simulink model "Master_Robot"  (R2019b)
settings: Solver=VariableStepAuto  StartTime=0.0  StopTime=10  RelTol=1e-3
undefined symbols (not defined in the file): Bh, Bs, Fc_h, Jh, k_m, Kc2v_m, Kd_h, Kd_s, Kp_h, Kp_s, Ks, Kt2c_m, lArm_m, maxCurrent_m, tau_s
settings Model: Creator=Mirko  LastModifiedBy=Mirko
settings SFSimCC: CustomCodeUndefinedFunction=UseInterfaceOnly

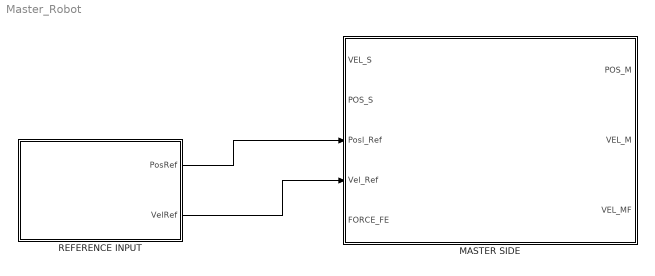
== system Master_Robot ==
  MASTER SIDE : Subsystem
  REFERENCE INPUT : Subsystem
  wires:
  REFERENCE INPUT/1(PosRef) -> MASTER SIDE/3(Posl_Ref)
  REFERENCE INPUT/2(VelRef) -> MASTER SIDE/4(Vel_Ref)

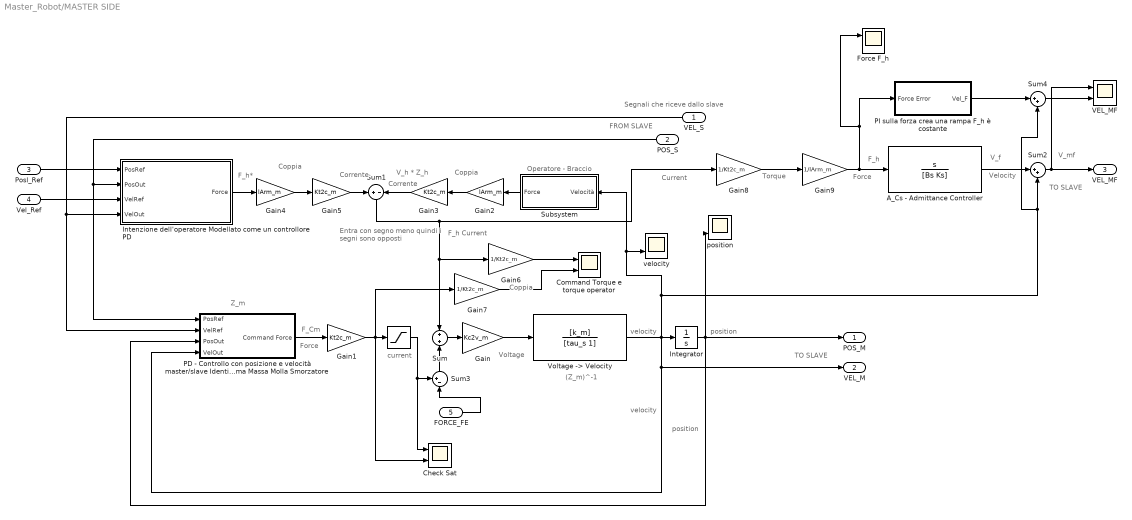
== system Master_Robot/MASTER SIDE ==
  note: Velocity
  note: Force
  note: Torque
  note: Current
  note: V_mf
  note: V_f
  note: F_h
  note: Z_m
  note: (Z_m)^-1
  note: F_h Current
  note: V_h * Z_h
  note: F_h*
  note: F_Cm
  note: FROM SLAVE
  note: TO SLAVE
  note: Coppia
  note: Entra con segno meno quindi
      | i segni sono opposti
  note: Corrente
  note: Coppia
  note: Corrente
  note: Coppia
  note: Segnali che riceve dallo slave
  note: Operatore - Braccio
  note: current
  note: Force
  note: Voltage
  note: position
  note: velocity
  note: position
  note: velocity
  note: TO SLAVE
  "VEL_S " : Inport
  POS_S : Inport  Port=2
  Posl_Ref : Inport  Port=3
  Vel_Ref : Inport  Port=4
  "FORCE_FE " : Inport  Port=5
  " " : Saturate  UpperLimit=maxCurrent_m  LowerLimit=-maxCurrent_m
  A_Cs - Admittance Controller : TransferFcn  Numerator=[1 0]  Denominator=[Bs Ks]
  Check Sat : Scope  NumInputPorts=2
  "Command Torque e torque operator " : Scope  NumInputPorts=2
  "Force F_h " : Scope  NumInputPorts=2
  Gain : Gain  Gain=Kc2v_m
  Gain1 : Gain  Gain=Kt2c_m
  Gain2 : Gain  Gain=lArm_m
  Gain3 : Gain  Gain=Kt2c_m
  Gain4 : Gain  Gain=lArm_m
  Gain5 : Gain  Gain=Kt2c_m
  Gain6 : Gain  Gain=1/Kt2c_m
  Gain7 : Gain  Gain=1/Kt2c_m
  Gain8 : Gain  Gain=1/Kt2c_m
  Gain9 : Gain  Gain=1/lArm_m
  Integrator : Integrator
  Intenzione dell'operatore Modellato come un controllore PD : Subsystem
  PD - Controllo con posizione e velocità master/slave Identico all'accoppiamento virtuale Sistema Massa Molla Smorzatore : Subsystem
  "PI sulla forza crea una rampa F_h è costante " : Subsystem
  Subsystem : Subsystem
  Sum : Sum
  Sum1 : Sum  Inputs=+-
  Sum2 : Sum  Inputs=|++
  Sum3 : Sum  Inputs=+-|
  Sum4 : Sum  Inputs=|++
  "VEL_MF " : Scope  NumInputPorts=2
  "Voltage -> Velocity " : TransferFcn  Numerator=[k_m]  Denominator=[tau_s 1]
  position : Scope  NumInputPorts=2
  velocity : Scope  NumInputPorts=2
  POS_M : Outport
  VEL_M : Outport  Port=2
  VEL_MF : Outport  Port=3
  wires:
  Gain1/1 -> Gain7/1, Check Sat/2, " "/1
  "VEL_S "/1 -> PD - Controllo con posizione e velocità master/slave Identico all'accoppiamento virtuale Sistema Massa Molla Smorzatore/2(VelRef), Intenzione dell'operatore Modellato come un controllore PD/4(VelOut)
  Integrator/1 -> PD - Controllo con posizione e velocità master/slave Identico all'accoppiamento virtuale Sistema Massa Molla Smorzatore/3(PosOut), position/2, POS_M/1
  ? -> position/1
  "Voltage -> Velocity "/1 -> PD - Controllo con posizione e velocità master/slave Identico all'accoppiamento virtuale Sistema Massa Molla Smorzatore/4(VelOut), VEL_M/1, Integrator/1, Sum4/2, Sum2/2, Subsystem/1("Velocità "), velocity/2
  Sum1/1 -> Gain8/1, Gain6/1, Sum/1
  Gain4/1 -> Gain5/1
  Gain6/1 -> "Command Torque e torque operator "/1
  Subsystem/1(Force) -> Gain2/1
  POS_S/1 -> Intenzione dell'operatore Modellato come un controllore PD/2(PosOut), PD - Controllo con posizione e velocità master/slave Identico all'accoppiamento virtuale Sistema Massa Molla Smorzatore/1(PosRef)
  Gain2/1 -> Gain3/1
  PD - Controllo con posizione e velocità master/slave Identico all'accoppiamento virtuale Sistema Massa Molla Smorzatore/1("Command Force ") -> Gain1/1
  Gain3/1 -> Sum1/2
  Gain7/1 -> "Command Torque e torque operator "/2
  Gain5/1 -> Sum1/1
  " "/1 -> Check Sat/1, Sum3/1
  ? -> velocity/1
  Intenzione dell'operatore Modellato come un controllore PD/1("Force ") -> Gain4/1
  Gain/1 -> "Voltage -> Velocity "/1
  Sum/1 -> Gain/1
  Posl_Ref/1 -> Intenzione dell'operatore Modellato come un controllore PD/1("PosRef ")
  Vel_Ref/1 -> Intenzione dell'operatore Modellato come un controllore PD/3(VelRef)
  A_Cs - Admittance Controller/1 -> Sum2/1
  Sum2/1 -> "VEL_MF "/1, VEL_MF/1
  "FORCE_FE "/1 -> Sum3/2
  Sum3/1 -> Sum/2
  Gain8/1 -> Gain9/1
  Gain9/1 -> "Force F_h "/1, "PI sulla forza crea una rampa F_h è costante "/1("Force Error "), A_Cs - Admittance Controller/1
  "PI sulla forza crea una rampa F_h è costante "/1(Vel_F) -> Sum4/1
  Sum4/1 -> "VEL_MF "/2

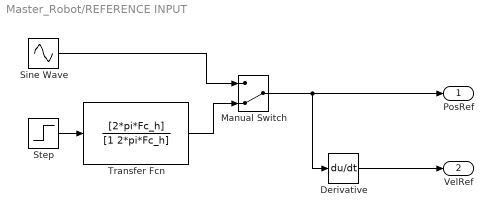
== system Master_Robot/REFERENCE INPUT ==
  Derivative : Derivative
  Manual Switch : ManualSwitch  CurrentSetting=0
  Sine Wave : Sin  SampleTime=0
  Step : Step  SampleTime=0
  Transfer Fcn : TransferFcn  Numerator=[2*pi*Fc_h]  Denominator=[1 2*pi*Fc_h]
  PosRef : Outport
  VelRef : Outport  Port=2
  wires:
  Sine Wave/1 -> Manual Switch/1
  Step/1 -> Transfer Fcn/1
  Transfer Fcn/1 -> Manual Switch/2
  Manual Switch/1 -> Derivative/1, PosRef/1
  Derivative/1 -> VelRef/1

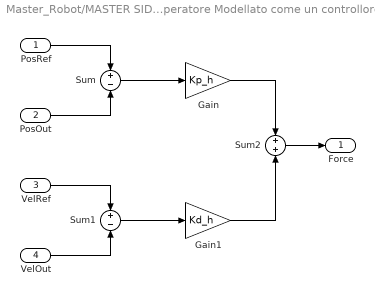
== system Master_Robot/MASTER SIDE/Intenzione dell'operatore Modellato come un controllore PD ==
  "PosRef " : Inport
  PosOut : Inport  Port=2
  VelRef : Inport  Port=3
  VelOut : Inport  Port=4
  Gain : Gain  Gain=Kp_h
  Gain1 : Gain  Gain=Kd_h
  Sum : Sum  Inputs=+-
  Sum1 : Sum  Inputs=+-
  Sum2 : Sum
  "Force " : Outport
  wires:
  PosOut/1 -> Sum/2
  "PosRef "/1 -> Sum/1
  Sum/1 -> Gain/1
  Sum1/1 -> Gain1/1
  VelRef/1 -> Sum1/1
  VelOut/1 -> Sum1/2
  Sum2/1 -> "Force "/1
  Gain1/1 -> Sum2/2
  Gain/1 -> Sum2/1

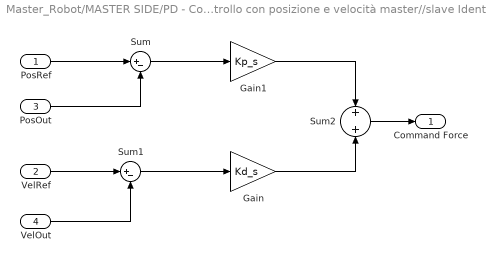
== system Master_Robot/MASTER SIDE/PD - Controllo con posizione e velocità master//slave Identico all'accoppiamento virtuale Sistema Massa Molla Smorzatore ==
  PosRef : Inport
  VelRef : Inport  Port=2
  PosOut : Inport  Port=3
  VelOut : Inport  Port=4
  Gain : Gain  Gain=Kd_s
  Gain1 : Gain  Gain=Kp_s
  Sum : Sum  Inputs=|+-
  Sum1 : Sum  Inputs=|+-
  Sum2 : Sum
  "Command Force " : Outport
  wires:
  PosRef/1 -> Sum/1
  PosOut/1 -> Sum/2
  VelRef/1 -> Sum1/1
  VelOut/1 -> Sum1/2
  Sum1/1 -> Gain/1
  Sum/1 -> Gain1/1
  Gain1/1 -> Sum2/1
  Gain/1 -> Sum2/2
  Sum2/1 -> "Command Force "/1

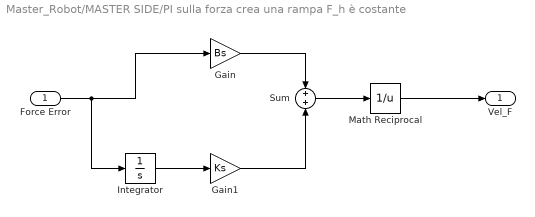
== system Master_Robot/MASTER SIDE/PI sulla forza crea una rampa F_h è costante  ==
  "Force Error " : Inport
  Gain : Gain  Gain=Bs
  Gain1 : Gain  Gain=Ks
  Integrator : Integrator
  Math Reciprocal : Math  Operator=reciprocal  SaturateOnIntegerOverflow=on
  Sum : Sum
  Vel_F : Outport
  wires:
  Gain/1 -> Sum/1
  Gain1/1 -> Sum/2
  "Force Error "/1 -> Integrator/1, Gain/1
  Integrator/1 -> Gain1/1
  Sum/1 -> Math Reciprocal/1
  Math Reciprocal/1 -> Vel_F/1

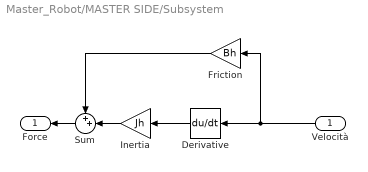
== system Master_Robot/MASTER SIDE/Subsystem ==
  "Velocità " : Inport
  Derivative : Derivative  CoefficientInTFapproximation=0.01
  Friction : Gain  Gain=Bh
  Inertia : Gain  Gain=Jh
  Sum : Sum  Inputs=++|
  Force : Outport
  wires:
  "Velocità "/1 -> Friction/1, Derivative/1
  Derivative/1 -> Inertia/1
  Inertia/1 -> Sum/2
  Friction/1 -> Sum/1
  Sum/1 -> Force/1
